simulink model "FMC_Ereg_Test"  (R2025a)
settings: Solver=daessc  StartTime=0.0  StopTime=stopTime  RelTol=1e-3
libraries: nesl_utility x1
settings Model: Creator=mu22504  LastModifiedBy=MW
settings DataIOCC: InspectSignalLogs=on
settings SimscapeCC: SimscapeLogType=all  SimscapeLogSimulationStatistics=on  SimscapeLogToSDI=on

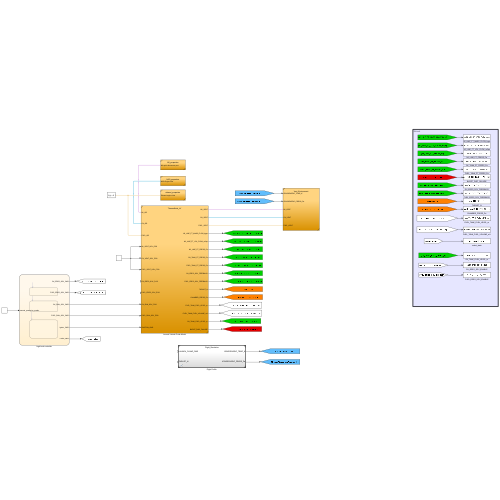
[thumbnail: Simulink's stored preview of the top-level diagram]
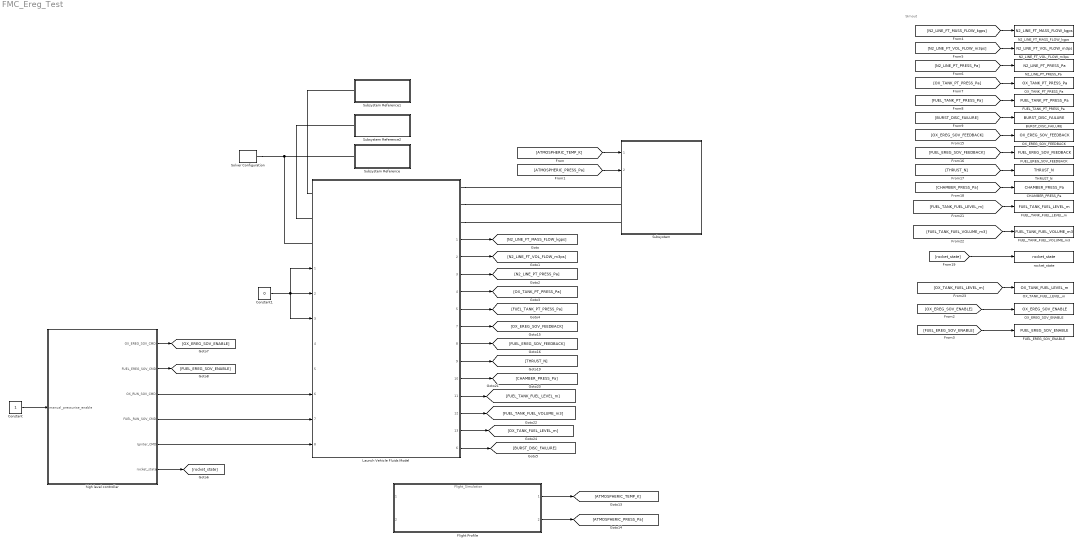
== system FMC_Ereg_Test ==
  note: SImout
  BURST_DISC_FAILURE : ToWorkspace  VariableName=BURST_DISC_FAILURE  SaveFormat=Timeseries  SampleTime=-1
  CHAMBER_PRESS_Pa : ToWorkspace  VariableName=CHAMBER_PRESS_Pa  SaveFormat=Timeseries  SampleTime=-1
  Constant : Constant
  Constant1 : Constant  Value=0
  FUEL_EREG_SOV_ENABLE : ToWorkspace  VariableName=FUEL_EREG_SOV_ENABLE  SaveFormat=Timeseries  SampleTime=-1
  FUEL_EREG_SOV_FEEDBACK : ToWorkspace  VariableName=FUEL_EREG_SOV_FEEDBACK  SaveFormat=Timeseries  SampleTime=-1
  FUEL_TANK_FUEL_LEVEL_m : ToWorkspace  VariableName=FUEL_TANK_FUEL_LEVEL_m  SaveFormat=Timeseries  SampleTime=-1
  FUEL_TANK_FUEL_VOLUME_m3 : ToWorkspace  VariableName=FUEL_TANK_FUEL_VOLUME_m3  SaveFormat=Timeseries  SampleTime=-1
  FUEL_TANK_PT_PRESS_Pa : ToWorkspace  VariableName=FUEL_TANK_PT_PRESS_Pa  SaveFormat=Timeseries  SampleTime=-1
  "Flight Profile " : ModelReference  ModelNameDialog=Flight_Simulation.slx  SimulationMode=Normal  ModelReferenceVersion=1.3
  Launch Vehicle Fluids Model : Subsystem  ReferencedSubsystem=Thermofluids_LV
      settings: PortSchema="{\"entries\":[{\"content\":{\"sides\":[{\"content\":{\"connectorIds\":[\"LConn1\",\"LConn2\",\"LConn6\",\"In1\",\"In2\",\"In3\",\"In4\",\"In5\",\"In6\",\"In7\",\"In8\"]},\"type\":\"ConnectorPlacement.EquallySpacedRectSide\",\"uuid\":\"a87b0425-c6b8-4d08-a1a8-b3acad5c334a\"},{\"content\":{\"connectorIds\":[\"LConn3\",\"LConn4\",\"LConn5\",\"Out1\",\"Out2\",\"Out3\",\"Out4\",\"Out5\",\"Out7\",\"Out8\",\"Out9\",\"Out10\",\"Out11\",\"Out12\",\"Out13\",\"Out6\"],\"side\":\"RIGHT\"},\"type\":\"ConnectorPlacement.EquallySpacedRectSide\",\"uuid\":\"260d6155-6d20-4ed3-9052-698506ea1559\"},{\"content\":{\"side\":\"TOP\"},\"type\":\"ConnectorPlacement.EquallySpacedRectSide\",\"uuid\":\"d266d02d-922b-4f41-b529-513bc445e931\"}]},\"type\":\"ConnectorPlacement.EquallySpacedConnector\",\"uuid\":\"36f51c95-b9e3-4232-bda9-d5a6ea8a2ffc\"}],\"packageUris\":[\"http://schema.mathworks.com/mf0/Connector/R2020b\"],\"version\":\"1.0\"}"
  N2_LINE_FT_MASS_FLOW_kgps : ToWorkspace  VariableName=N2_LINE_FT_MASS_FLOW_kgps  SaveFormat=Timeseries  SampleTime=-1
  N2_LINE_FT_VOL_FLOW_m3ps : ToWorkspace  VariableName=N2_LINE_FT_VOL_FLOW_m3ps  SaveFormat=Timeseries  SampleTime=-1
  N2_LINE_PT_PRESS_Pa : ToWorkspace  VariableName=N2_LINE_PT_PRESS_Pa  SaveFormat=Timeseries  SampleTime=-1
  OX_EREG_SOV_ENABLE : ToWorkspace  VariableName=OX_EREG_SOV_ENABLE  SaveFormat=Timeseries  SampleTime=-1
  OX_EREG_SOV_FEEDBACK : ToWorkspace  VariableName=OX_EREG_SOV_FEEDBACK  SaveFormat=Timeseries  SampleTime=-1
  OX_TANK_FUEL_LEVEL_m : ToWorkspace  VariableName=OX_TANK_FUEL_LEVEL_m  SaveFormat=Timeseries  SampleTime=-1
  OX_TANK_PT_PRESS_Pa : ToWorkspace  VariableName=OX_TANK_PT_PRESS_Pa  SaveFormat=Timeseries  SampleTime=-1
  Solver Configuration : nesl_utility/Solver Configuration  PhysicalDomain=network_engine_domain  SubClassName=solver  LeftPortType=input  RightPortType=generic  Tones=[]  Harmonics=[]  SimulateNoise=off  Profile=off  UseLocalSampling=off  EnableSwitchedLinearOptims=on  FrequencyDomain=off  UseCCode=off  RelTol=0.001  AbsTol=0.001  MinStep=1e-09  ToWorkspace=off  RevertToSquareIcSolve=off  NumHomotopyIterations=100  PhasorMode=off  PhasorModeNumHarmonics=1  ConsistencySolver=NEWTON_XTOL_AFTER_FTOL  IndexReductionMethod=DerivativeReplacement  DoDC=off  ResidualTolerance=1e-09  ConsistencyTolSource=GLOBAL  ConsistencyAbsTol=0.001  ConsistencyRelTol=0.001  ConsistencyTolFactor=0.001  UseLocalSolver=off  LocalSolverChoice=NE_BACKWARD_EULER_ADVANCER  ResolveIndetEquations=on  FunctionEvalNumThread=1  LocalSolverSampleTime=0.001  DoFixedCost=off  MaxNonlinIter=3  MaxModeIter=2  ComputeImpulses=off  ImpulseIterations=2  LinearAlgebra=auto  LinearAlgebraNumThread=0  EquationFormulation=NE_TIME_EF  DelaysMemoryBudget=1024  AutomaticFiltering=on  FilteringTimeConstant=0.001  PartitionStorageMethod=AS_NEEDED  PartitionMemoryBudget=1024  PartitionMethod=ROBUST  MultibodyUseLocalSolver=off  MultibodyLocalSolverChoice=ODE1  MultibodyLocalSolverSampleTime=0.001
  Subsystem : Subsystem  ReferencedSubsystem=Vent_Environment
  Subsystem Reference : Subsystem  ReferencedSubsystem=ethanol_properties
  Subsystem Reference1 : Subsystem  ReferencedSubsystem=N2_properties
  Subsystem Reference2 : Subsystem  ReferencedSubsystem=N2O_properties
  THRUST_N : ToWorkspace  VariableName=THRUST_N  SaveFormat=Timeseries  SampleTime=-1
  high level controller : Stateflow chart  TreatAsAtomicUnit=on
  rocket_state : ToWorkspace  VariableName=rocket_state  SaveFormat=Timeseries  SampleTime=-1
  wires:
  [N2_LINE_FT_MASS_FLOW_kgps] -> N2_LINE_FT_MASS_FLOW_kgps/1
  [BURST_DISC_FAILURE] -> BURST_DISC_FAILURE/1
  [FUEL_TANK_PT_PRESS_Pa] -> FUEL_TANK_PT_PRESS_Pa/1
  [OX_TANK_PT_PRESS_Pa] -> OX_TANK_PT_PRESS_Pa/1
  [N2_LINE_PT_PRESS_Pa] -> N2_LINE_PT_PRESS_Pa/1
  [N2_LINE_FT_VOL_FLOW_m3ps] -> N2_LINE_FT_VOL_FLOW_m3ps/1
  [OX_EREG_SOV_FEEDBACK] -> OX_EREG_SOV_FEEDBACK/1
  [FUEL_EREG_SOV_FEEDBACK] -> FUEL_EREG_SOV_FEEDBACK/1
  [THRUST_N] -> THRUST_N/1
  [CHAMBER_PRESS_Pa] -> CHAMBER_PRESS_Pa/1
  [FUEL_TANK_FUEL_VOLUME_m3] -> FUEL_TANK_FUEL_VOLUME_m3/1
  [FUEL_TANK_FUEL_LEVEL_m] -> FUEL_TANK_FUEL_LEVEL_m/1
  [rocket_state] -> rocket_state/1
  [OX_TANK_FUEL_LEVEL_m] -> OX_TANK_FUEL_LEVEL_m/1
  Launch Vehicle Fluids Model/10 -> [CHAMBER_PRESS_Pa]
  Launch Vehicle Fluids Model/11 -> [FUEL_TANK_FUEL_LEVEL_m]
  Launch Vehicle Fluids Model/6 -> [BURST_DISC_FAILURE]
  Launch Vehicle Fluids Model/4 -> [OX_TANK_PT_PRESS_Pa]
  Launch Vehicle Fluids Model/3 -> [N2_LINE_PT_PRESS_Pa]
  Launch Vehicle Fluids Model/5 -> [FUEL_TANK_PT_PRESS_Pa]
  Launch Vehicle Fluids Model/13 -> [OX_TANK_FUEL_LEVEL_m]
  Launch Vehicle Fluids Model/1 -> [N2_LINE_FT_MASS_FLOW_kgps]
  Launch Vehicle Fluids Model/2 -> [N2_LINE_FT_VOL_FLOW_m3ps]
  Launch Vehicle Fluids Model/9 -> [THRUST_N]
  Launch Vehicle Fluids Model/12 -> [FUEL_TANK_FUEL_VOLUME_m3]
  Launch Vehicle Fluids Model/7 -> [OX_EREG_SOV_FEEDBACK]
  Launch Vehicle Fluids Model/8 -> [FUEL_EREG_SOV_FEEDBACK]
  "Flight Profile "/1 -> [ATMOSPHERIC_TEMP_K]
  "Flight Profile "/2 -> [ATMOSPHERIC_PRESS_Pa]
  [ATMOSPHERIC_TEMP_K] -> Subsystem/1
  [ATMOSPHERIC_PRESS_Pa] -> Subsystem/2
  Constant/1 -> high level controller/1(manual_pressurise_enable)
  Constant1/1 -> Launch Vehicle Fluids Model/2, Launch Vehicle Fluids Model/3, Launch Vehicle Fluids Model/1
  high level controller/3(OX_RUN_SOV_CMD) -> Launch Vehicle Fluids Model/6
  high level controller/4(FUEL_RUN_SOV_CMD) -> Launch Vehicle Fluids Model/7
  high level controller/5(Igniter_CMD) -> Launch Vehicle Fluids Model/8
  high level controller/6(rocket_state) -> [rocket_state]
  high level controller/1(OX_EREG_SOV_CMD) -> [OX_EREG_SOV_ENABLE]
  high level controller/2(FUEL_EREG_SOV_CMD) -> [FUEL_EREG_SOV_ENABLE]
  [OX_EREG_SOV_ENABLE] -> OX_EREG_SOV_ENABLE/1
  [FUEL_EREG_SOV_ENABLE] -> FUEL_EREG_SOV_ENABLE/1
  connections:
  Launch Vehicle Fluids Model/LConn6 -- Solver Configuration/RConn1 -- Subsystem Reference/LConn1
  Subsystem Reference2/LConn1 -- Launch Vehicle Fluids Model/LConn2
  Subsystem Reference1/LConn1 -- Launch Vehicle Fluids Model/LConn1
  Launch Vehicle Fluids Model/LConn3 -- Subsystem/LConn1
  Launch Vehicle Fluids Model/LConn4 -- Subsystem/LConn2
  Launch Vehicle Fluids Model/LConn5 -- Subsystem/LConn3

== stateflow chart FMC_Ereg_Test/high level controller ==
  state Manual_Pressurisation_WAIT
    en:
    rocket_state = 6;
  state Ignition_precondition
    en:
    rocket_state = 7;
    OX_EREG_SOV_CMD = 1;
    FUEL_EREG_SOV_CMD = 1;
  state Launch
    en:
    rocket_state = 8;
    OX_RUN_SOV_CMD = 1;
    FUEL_RUN_SOV_CMD = 1;
    Igniter_CMD = 1;
  (default) -> Manual_Pressurisation_WAIT
  Manual_Pressurisation_WAIT -> Ignition_precondition : [manual_pressurise_enable == 1]
  Ignition_precondition -> Launch : after(10, sec)
  data: OX_EREG_SOV_CMD output; manual_pressurise_enable input; FUEL_EREG_SOV_CMD output; OX_RUN_SOV_CMD output; FUEL_RUN_SOV_CMD output; Igniter_CMD output; rocket_state output
